simulink model "kalman_with_testbench_for_vivado"  (R2026a)
settings: Solver=ode3  StopTime=5  FixedStep=0.00001
libraries: fl_lib x4, nesl_utility x3, simulink x1, ee_lib x1
settings Model: Creator=eipek  LastModifiedBy=eipek
settings OptimizationCC: ConditionallyExecuteInputs=off
settings DebuggingCC: SignalRangeChecking=warning  AlgebraicLoopMsg=error
settings HardwareCC: ProdHWDeviceType=ASIC/FPGA->ASIC/FPGA  TargetBitPerPointer=64.0  TargetBitPerSizeT=64.0  TargetBitPerPtrDiffT=64.0  TargetLongLongMode=on  TargetIntDivRoundTo=Zero  TargetEndianess=LittleEndian  TargetWordSize=64.0  TargetHWDeviceType=Custom Processor->MATLAB Host Computer  ProdEqTarget=off
settings SimscapeCC: SimscapeNominalValues="[{\"value\":\"1\",\"unit\":\"A\"},{\"value\":\"1\",\"unit\":\"bar\"},{\"value\":\"1\",\"unit\":\"cm^2\"},{\"value\":\"1\",\"unit\":\"cm^3/s\"},{\"value\":\"1\",\"unit\":\"kJ/kg\"},{\"value\":\"1\",\"unit\":\"kW\"},{\"value\":\"1\",\"unit\":\"l\"},{\"value\":\"1\",\"unit\":\"N\"},{\"value\":\"1\",\"unit\":\"N*m\"},{\"value\":\"1\",\"unit\":\"V\"}]"  SimscapeLogType=none  SimscapeLogDataHistory=5000.0

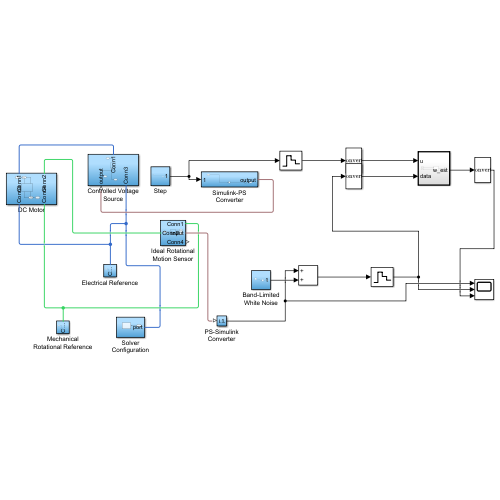
[thumbnail: Simulink's stored preview of the top-level diagram]
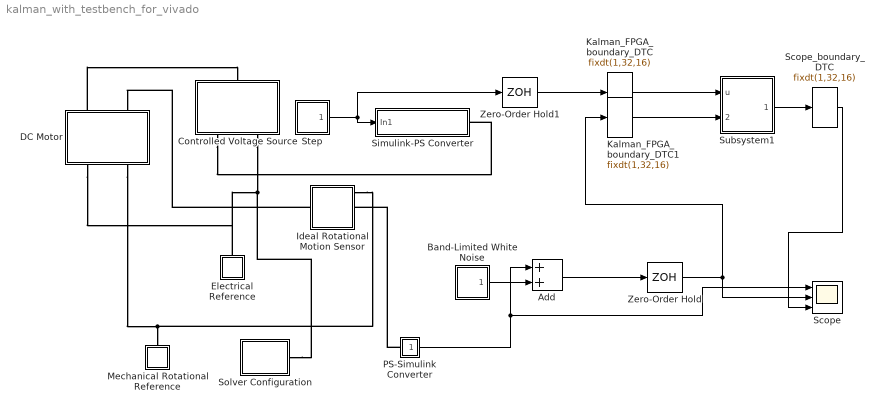
== system kalman_with_testbench_for_vivado ==
  Add : Sum
  Band-Limited White Noise : Subsystem  Tag=DecoupledSystem
  Controlled Voltage Source : Subsystem  Tag=DecoupledSystem
  DC Motor : Subsystem  Tag=DecoupledSystem
  Electrical Reference : Subsystem  Tag=DecoupledSystem
  Ideal Rotational Motion Sensor : Subsystem  Tag=DecoupledSystem
  Kalman_FPGA_boundary_DTC : DataTypeConversion  OutDataTypeStr=fixdt(1,32,16)
  Kalman_FPGA_boundary_DTC1 : DataTypeConversion  OutDataTypeStr=fixdt(1,32,16)
  Mechanical Rotational Reference : Subsystem  Tag=DecoupledSystem
  PS-Simulink Converter : Subsystem  Tag=DecoupledSystem
  Scope : Scope  NumInputPorts=3
      settings: ActiveDisplayYMinimum=51.180262823785419  ActiveDisplayYMaximum=111.74758317479646
  Scope_boundary_DTC : DataTypeConversion  OutDataTypeStr=fixdt(1,32,16)
  Simulink-PS Converter : Subsystem  Tag=DecoupledSystem
  Solver Configuration : Subsystem  Tag=DecoupledSystem
  Step : Subsystem  Tag=DecoupledSystem
  Subsystem1 : Subsystem  TreatAsAtomicUnit=on  SystemSampleTime=0.01
  Zero-Order Hold : ZeroOrderHold  SampleTime=0.01
  Zero-Order Hold1 : ZeroOrderHold  SampleTime=0.01
  wires:
  Step/1(Out1) -> Zero-Order Hold1/1, Simulink-PS Converter/1(In1)
  PS-Simulink Converter/1(Out1) -> Add/1, Scope/1
  Band-Limited White Noise/1(Out1) -> Add/2
  Add/1 -> Zero-Order Hold/1
  Zero-Order Hold/1 -> Kalman_FPGA_boundary_DTC1/1, Scope/2
  Scope_boundary_DTC/1 -> Scope/3
  Kalman_FPGA_boundary_DTC/1 -> Subsystem1/1(u)
  Kalman_FPGA_boundary_DTC1/1 -> Subsystem1/2(data)
  Subsystem1/1(w_est) -> Scope_boundary_DTC/1
  Zero-Order Hold1/1 -> Kalman_FPGA_boundary_DTC/1
  connections:
  Controlled Voltage Source/RConn2 -- Electrical Reference/LConn1 -- DC Motor/RConn1 -- Solver Configuration/RConn1
  DC Motor/LConn1 -- Controlled Voltage Source/LConn1
  Controlled Voltage Source/RConn1 -- Simulink-PS Converter/RConn1
  DC Motor/RConn2 -- Mechanical Rotational Reference/LConn1 -- Ideal Rotational Motion Sensor/RConn1
  Ideal Rotational Motion Sensor/LConn1 -- DC Motor/LConn2
  PS-Simulink Converter/LConn1 -- Ideal Rotational Motion Sensor/RConn2

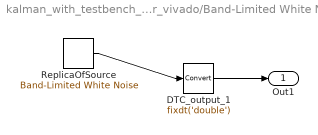
== system kalman_with_testbench_for_vivado/Band-Limited White Noise ==
  DTC_output_1 : DataTypeConversion  OutDataTypeStr=fixdt('double')  SaturateOnIntegerOverflow=off  RndMeth=Floor
  ReplicaOfSource : simulink/Sources/Band-Limited White Noise  Cov=0.005  Ts=0.001  seed=[23341]
  Out1 : Outport  LockScale=on
  wires:
  DTC_output_1/1 -> Out1/1
  ReplicaOfSource/1 -> DTC_output_1/1

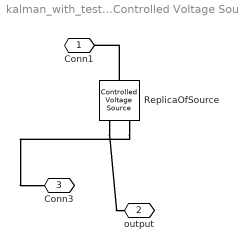
== system kalman_with_testbench_for_vivado/Controlled Voltage Source ==
  ReplicaOfSource : fl_lib/Electrical/Electrical Sources/Controlled Voltage Source
  Conn1 : PMIOPort  Side=Left
  output : PMIOPort  Port=2  Side=Right
  Conn3 : PMIOPort  Port=3  Side=Right
  connections:
  ReplicaOfSource/RConn2 -- Conn3/RConn1
  ReplicaOfSource/RConn1 -- output/RConn1
  ReplicaOfSource/LConn1 -- Conn1/RConn1

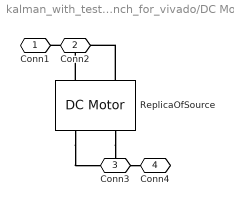
== system kalman_with_testbench_for_vivado/DC Motor ==
  ReplicaOfSource : ee_lib/Electromechanical/Brushed Motors/DC Motor  field_option=ee.enum.field_option.pm  Rf=100 Ohm  Lf=1 H  Laf=0.15 H  If0=0 A  parameterization=ee.enum.dcparam_option.circuit_param  Ra=15 Ohm  La=0.015 H  emf_or_torque=ee.enum.emf_or_torque.kv  Kv=0.086 V*s/rad  Ki=6.876e-4 N*m/A  T_stall=0.24e-3 N*m  w_max=19100 rpm  w_rated=15000 rpm  P_rated=0.08 W  V_rated=1.5 V  lam_param=ee.enum.lam_param.damping  i_noload=0 A  V_i_noload=1.5 V  J=9.86e-6 kg*m^2  lam=1.64e-4 N*m*s/rad  speed0=0 rpm  alpha=3.93e-3 1/K  Tmeas=25 degC  thermal_mass=100 J/K  initial_temperature=25 degC
  Conn1 : PMIOPort  Side=Left
  Conn2 : PMIOPort  Port=2  Side=Left
  Conn3 : PMIOPort  Port=3  Side=Right
  Conn4 : PMIOPort  Port=4  Side=Right
  connections:
  ReplicaOfSource/LConn1 -- Conn1/RConn1
  ReplicaOfSource/RConn2 -- Conn4/RConn1
  ReplicaOfSource/LConn2 -- Conn2/RConn1
  ReplicaOfSource/RConn1 -- Conn3/RConn1

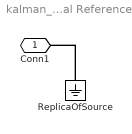
== system kalman_with_testbench_for_vivado/Electrical Reference ==
  ReplicaOfSource : fl_lib/Electrical/Electrical Elements/Electrical Reference
  Conn1 : PMIOPort  Side=Left
  connections:
  ReplicaOfSource/LConn1 -- Conn1/RConn1

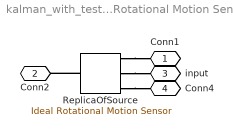
== system kalman_with_testbench_for_vivado/Ideal Rotational Motion Sensor ==
  ReplicaOfSource : fl_lib/Mechanical/Mechanical Sensors/Ideal Rotational Motion Sensor  reference=foundation.enum.MeasurementReference.difference  acceleration_port=false  velocity_port=true  position_port=true  wrap_angle=false  offset=0 rad
  Conn1 : PMIOPort  Side=Right
  Conn2 : PMIOPort  Port=2  Side=Left
  input : PMIOPort  Port=3  Side=Right
  Conn4 : PMIOPort  Port=4  Side=Right
  connections:
  ReplicaOfSource/RConn1 -- Conn1/RConn1
  ReplicaOfSource/RConn3 -- Conn4/RConn1
  ReplicaOfSource/RConn2 -- input/RConn1
  ReplicaOfSource/LConn1 -- Conn2/RConn1

== system kalman_with_testbench_for_vivado/Mechanical Rotational Reference ==
  ReplicaOfSource : fl_lib/Mechanical/Rotational Elements/Mechanical Rotational Reference
  Conn1 : PMIOPort  Side=Left
  connections:
  ReplicaOfSource/LConn1 -- Conn1/RConn1

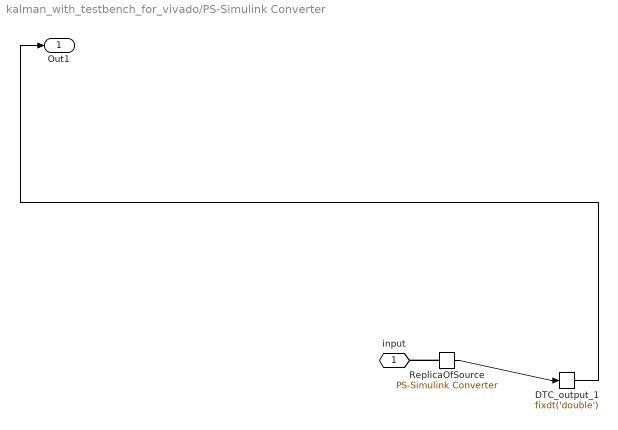
== system kalman_with_testbench_for_vivado/PS-Simulink Converter ==
  DTC_output_1 : DataTypeConversion  OutDataTypeStr=fixdt('double')  SaturateOnIntegerOverflow=off  RndMeth=Floor
  ReplicaOfSource : nesl_utility/PS-Simulink Converter  PhysicalDomain=network_engine_domain  SubClassName=ps_output  LeftPortType=input  RightPortType=output  PseudoPeriodic=off  Frequencies=[]  VectorFormat=inherit  Unit=inherit  AffineConversion=off
  input : PMIOPort  Side=Left
  Out1 : Outport  LockScale=on
  wires:
  DTC_output_1/1 -> Out1/1
  ReplicaOfSource/1 -> DTC_output_1/1
  connections:
  ReplicaOfSource/LConn1 -- input/RConn1

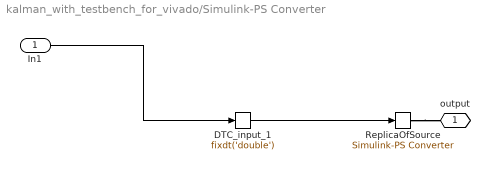
== system kalman_with_testbench_for_vivado/Simulink-PS Converter ==
  In1 : Inport  LockScale=on
  DTC_input_1 : DataTypeConversion  OutDataTypeStr=fixdt('double')  RndMeth=Nearest  SaturateOnIntegerOverflow=off  LockScale=on
  ReplicaOfSource : nesl_utility/Simulink-PS Converter  PhysicalDomain=network_engine_domain  SubClassName=ps_input  LeftPortType=input  RightPortType=output  PseudoPeriodic=off  Frequencies=[]  NoiseDistribution=none  NoiseParameters=[]  Unit=1  AffineConversion=off  FilteringAndDerivatives=provide  SimscapeFilterOrder=1  InputFilterTimeConstant=0.001  UdotUserProvided=0
  output : PMIOPort  Side=Right
  wires:
  In1/1 -> DTC_input_1/1
  DTC_input_1/1 -> ReplicaOfSource/1
  connections:
  ReplicaOfSource/RConn1 -- output/RConn1

== system kalman_with_testbench_for_vivado/Solver Configuration ==
  ReplicaOfSource : nesl_utility/Solver Configuration  PhysicalDomain=network_engine_domain  SubClassName=solver  LeftPortType=input  RightPortType=generic  Tones=[]  Harmonics=[]  SimulateNoise=off  Profile=off  UseLocalSampling=off  EnableSwitchedLinearOptims=on  FrequencyDomain=off  UseCCode=off  RelTol=0.001  AbsTol=0.001  MinStep=1e-09  ToWorkspace=off  RevertToSquareIcSolve=off  NumHomotopyIterations=100  PhasorMode=off  PhasorModeNumHarmonics=1  ConsistencySolver=NEWTON_XTOL_AFTER_FTOL  CanonicalOrdering=UNORDERED  OptimizeIntermediates=UNOPTIMIZED  IndexReductionMethod=DerivativeReplacement  DoDC=off  ResidualTolerance=1e-09  ConsistencyTolSource=GLOBAL  ConsistencyAbsTol=0.001  ConsistencyRelTol=0.001  ConsistencyTolFactor=0.001  UseLocalSolver=on  LocalSolverChoice=NE_BACKWARD_EULER_ADVANCER  ResolveIndetEquations=on  FunctionEvalNumThread=1  LocalSolverSampleTime=0.0001  DoFixedCost=off  MaxNonlinIter=3  MaxModeIter=2  ComputeImpulses=off  ImpulseIterations=2  LinearAlgebra=auto  LinearAlgebraNumThread=0  EquationFormulation=NE_TIME_EF  DelaysMemoryBudget=1024  AutomaticFiltering=on  FilteringTimeConstant=0.001  PartitionStorageMethod=AS_NEEDED  PartitionMemoryBudget=1024  PartitionMethod=ROBUST  MultibodyUseLocalSolver=off  MultibodyLocalSolverChoice=ODE1  MultibodyLocalSolverSampleTime=0.001
  port : PMIOPort  Side=Right
  connections:
  ReplicaOfSource/RConn1 -- port/RConn1

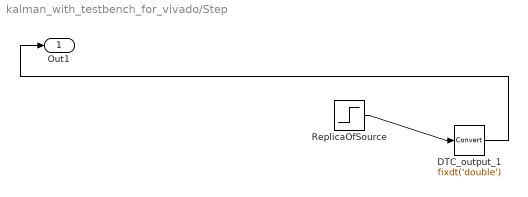
== system kalman_with_testbench_for_vivado/Step ==
  DTC_output_1 : DataTypeConversion  OutDataTypeStr=fixdt('double')  SaturateOnIntegerOverflow=off  RndMeth=Floor
  ReplicaOfSource : Step  Time=0.1  FinalValue=12  SampleTime=0
  Out1 : Outport  LockScale=on
  wires:
  ReplicaOfSource/1 -> DTC_output_1/1
  DTC_output_1/1 -> Out1/1

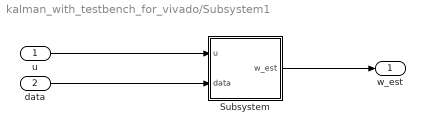
== system kalman_with_testbench_for_vivado/Subsystem1 ==
  u : Inport  OutDataTypeStr=fixdt(1,32,16)
  data : Inport  Port=2  OutDataTypeStr=fixdt(1,32,16)
  Subsystem : Subsystem
  w_est : Outport  OutDataTypeStr=fixdt(1,32,16)
  wires:
  u/1 -> Subsystem/1(u)
  Subsystem/1(w_est) -> w_est/1
  data/1 -> Subsystem/2(data)

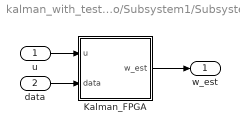
== system kalman_with_testbench_for_vivado/Subsystem1/Subsystem ==
  u : Inport
  data : Inport  Port=2
  Kalman_FPGA : Subsystem
  w_est : Outport
  wires:
  data/1 -> Kalman_FPGA/2(data)
  Kalman_FPGA/1(w_est) -> w_est/1
  u/1 -> Kalman_FPGA/1(u)

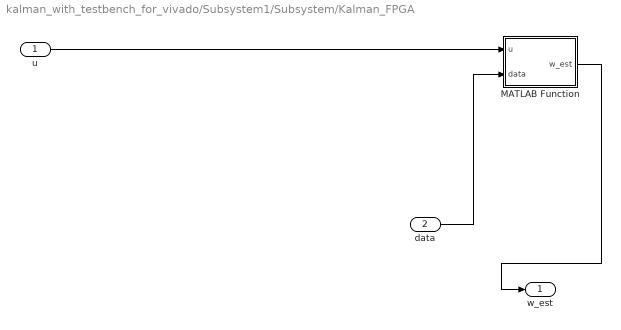
== system kalman_with_testbench_for_vivado/Subsystem1/Subsystem/Kalman_FPGA ==
  u : Inport
  data : Inport  Port=2
  MATLAB Function : MATLAB Function  TreatAsAtomicUnit=on
  w_est : Outport
  wires:
  MATLAB Function/1(w_est) -> w_est/1
  u/1 -> MATLAB Function/1(u)
  data/1 -> MATLAB Function/2(data)

== matlab function kalman_with_testbench_for_vivado/Subsystem1/Subsystem/Kalman_FPGA/MATLAB Function ==
  settings: updateMethod=DISCRETE
  data: u input; data input; w_est output
function w_est = fcn(u, data)

T = numerictype(1, 32, 16); 
F = fimath('RoundingMethod', 'Zero', 'OverflowAction', 'Saturate');

persistent x_est P R_k Ad Bd Cd Q alpha R0 Ad_t Cd_t I initialized

if isempty(initialized)

    Ad = fi([0.8500, 0.2000; -0.0100, 0.4000], T, F);
    Bd = fi([1.3050; 0.1000], T, F); 
    Cd = fi([1, 0], T, F); 

    Ad_t = fi([0.8500, -0.0100; 0.2000, 0.4000], T, F);
    Cd_t = fi([1; 0], T, F);
    I = fi([1 0; 0 1], T, F);
    
    x_est = fi([0; 0], T, F);

    P = fi([5.0, 0; 0, 20.0], T, F);
    
    Q = fi([0.2, 0; 0, 0.2], T, F);

    R0 = fi(5.0, T, F);
    alpha = fi(0.02, T, F);
    R_k = fi(5.0, T, F); 
    
    initialized = 1;
end


x_pred = fi(Ad * x_est + Bd * u, T, F);

P_pred = fi(Ad * P * Ad_t + Q, T, F);


y_pred = fi(Cd * x_pred, T, F);


residual = fi(data - y_pred, T, F);


R_k = fi(R0 + fi(alpha * abs(residual), T, F), T, F);


if R_k < fi(0.1, T, F)
    R_k = fi(0.1, T, F);
elseif R_k > fi(20.0, T, F)
    R_k = fi(20.0, T, F);
end

S_k = fi(fi(Cd * P_pred * Cd_t, T, F) + R_k, T, F);


if abs(S_k) < fi(0.001, T, F)
    K = fi([0; 0], T, F);
else
    K = fi((P_pred * Cd_t) / S_k, T, F);
end


x_est = fi(x_pred + fi(K * residual, T, F), T, F);


P = fi(fi(I - fi(K * Cd, T, F), T, F) * P_pred, T, F);


P12 = fi((P(1,2) + P(2,1)) / 2, T, F);
P(1,2) = P12;
P(2,1) = P12;


if P(1,1) < fi(0.0001, T, F)
    P(1,1) = fi(0.0001, T, F);
end

if P(2,2) < fi(0.0001, T, F)
    P(2,2) = fi(0.0001, T, F);
end


w_est = x_est(1);

end
